simulink model "lab2s"  (R2020b)
settings: Solver=VariableStepAuto  StartTime=0.0  StopTime=150.0  RelTol=1e-3
values from neighbouring files (symbols this model uses):
  A1 = pi .* R1 .^ 2    [lab2.m]
  A2 = pi * (R2 ^ 2)    (= 27.9999876063)    [lab2.m]
  C1 = 4.12311    [lab2.m]
  C2 = 2.91548    [lab2.m]
  h10 = (q10 / C1) .^ 2    [lab2.m]
  H2 = 17    [lab2.m]
  h20 = 1/2 .* H2    [lab2.m]
  q10 = C2 * sqrt(H2/2)    [lab2.m]
undefined symbols (not defined in the file or in its folder): x, x1, x2, y, y1, y2
settings Model: Creator=superstudent  LastModifiedBy=Marek
settings DataIOCC: ReturnWorkspaceOutputs=off
settings DebuggingCC: ArithmeticOperatorsInVariantConditions=warning
settings SFSimCC: SimUseLocalCustomCode=off  CustomCodeUndefinedFunction=UseInterfaceOnly
settings RTWCC: RTWUseLocalCustomCode=off
settings CodeAppCC: StateflowObjectComments=on

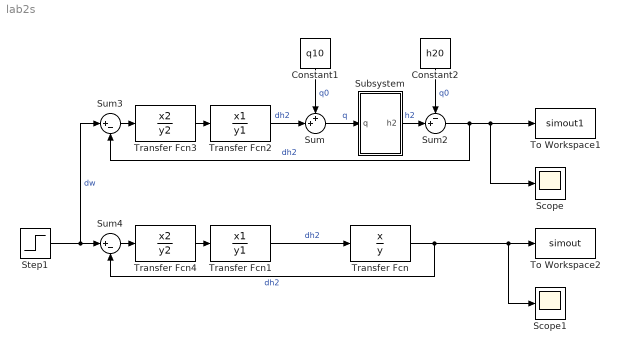
== system lab2s ==
  Constant1 : Constant  Value=q10
  Constant2 : Constant  Value=h20
  Scope : Scope
  Scope1 : Scope
  Step1 : Step  Time=0  SampleTime=0
  Subsystem : Subsystem
  Sum : Sum  Inputs=++|
  Sum2 : Sum  Inputs=-+|
  Sum3 : Sum  Inputs=|+-
  Sum4 : Sum  Inputs=|+-
  To Workspace1 : ToWorkspace  VariableName=simout1  SampleTime=-1
  To Workspace2 : ToWorkspace  VariableName=simout  SampleTime=-1
  Transfer Fcn : TransferFcn  Numerator=x  Denominator=y
  Transfer Fcn1 : TransferFcn  Numerator=x1  Denominator=y1
  Transfer Fcn2 : TransferFcn  Numerator=x1  Denominator=y1
  Transfer Fcn3 : TransferFcn  Numerator=x2  Denominator=y2
  Transfer Fcn4 : TransferFcn  Numerator=x2  Denominator=y2
  wires:
  Transfer Fcn/1 -> Scope1/1, To Workspace2/1, Sum4/2  "dh2"
  Transfer Fcn1/1 -> Transfer Fcn/1  "dh2"
  Transfer Fcn4/1 -> Transfer Fcn1/1
  Transfer Fcn3/1 -> Transfer Fcn2/1
  Transfer Fcn2/1 -> Sum/2  "dh2"
  Sum/1 -> Subsystem/1(q)  "q"
  Constant1/1 -> Sum/1  "q0"
  Constant2/1 -> Sum2/1  "q0"
  Subsystem/1(h2) -> Sum2/2  "h2"
  Sum2/1 -> Sum3/2, Scope/1, To Workspace1/1  "dh2"
  Sum3/1 -> Transfer Fcn3/1
  Sum4/1 -> Transfer Fcn4/1
  Step1/1 -> Sum3/1, Sum4/1  "dw"

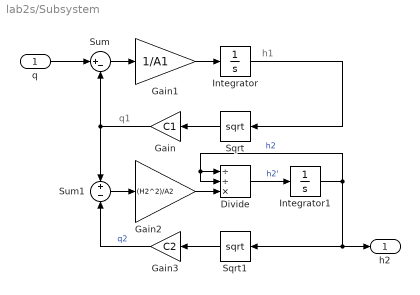
== system lab2s/Subsystem ==
  note: h1
  note: q1
  q : Inport
  Divide : Product  Inputs=//*
  Gain : Gain  Gain=C1
  Gain1 : Gain  Gain=1/A1
  Gain2 : Gain  Gain=(H2^2)/A2
  Gain3 : Gain  Gain=C2
  Integrator : Integrator  InitialCondition=h10
  Integrator1 : Integrator  InitialCondition=h20
  Sqrt : Sqrt  SaturateOnIntegerOverflow=on
  Sqrt1 : Sqrt  SaturateOnIntegerOverflow=on
  Sum : Sum  Inputs=|+-
  Sum1 : Sum  Inputs=+|-
  h2 : Outport
  wires:
  Gain/1 -> Sum1/1, Sum/2
  Sum/1 -> Gain1/1
  Sqrt1/1 -> Gain3/1
  Integrator1/1 -> h2/1, Sqrt1/1, Divide/1, Divide/2  "h2"
  Gain3/1 -> Sum1/2  "q2"
  Divide/1 -> Integrator1/1  "h2'"
  Integrator/1 -> Sqrt/1
  Sum1/1 -> Gain2/1
  Gain1/1 -> Integrator/1
  Sqrt/1 -> Gain/1
  Gain2/1 -> Divide/3
  q/1 -> Sum/1
